simulink model "band_pass_filter_cosim"  (Simulink 6.0)
settings: Solver=ode45  StartTime=0.0  StopTime=0.35  RelTol=1e-3
undefined symbols (not defined in the file): sigbuilder_block
libraries: aldec_ahdl x6
settings Model: LastModifiedBy=arekg

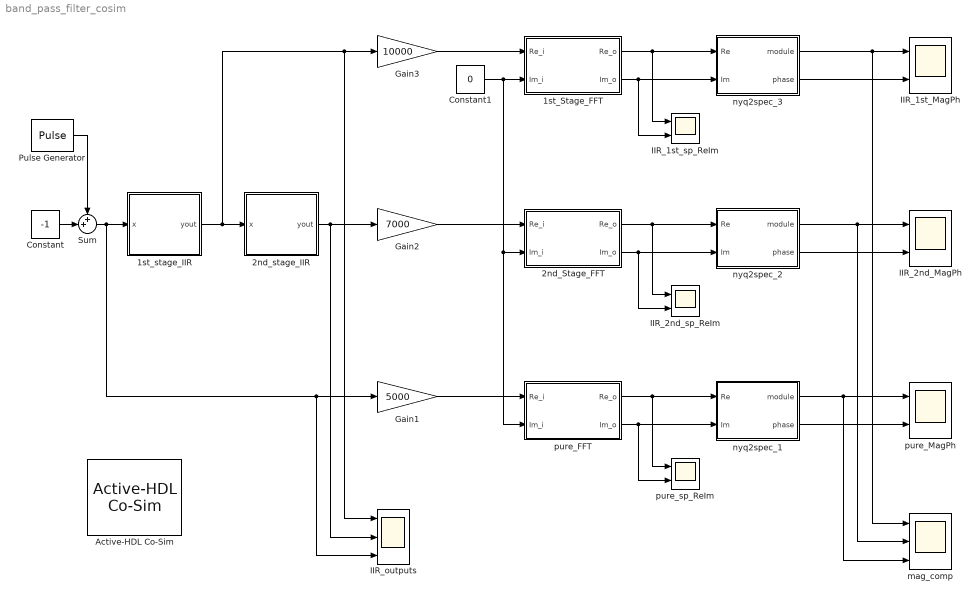
== system band_pass_filter_cosim ==
  1st_Stage_FFT : Subsystem
  1st_stage_IIR : Subsystem
  2nd_Stage_FFT : Subsystem
  2nd_stage_IIR : Subsystem
  Active-HDL Co-Sim : aldec_ahdl/Active-HDL Co-Sim  b_type=0  sys_period=1/88000  dbg=off  quit_en=off  gen_tb=off  tb_fn=mlab_post_tb.log
  Constant : Constant  Value=-1
  Constant1 : Constant  Value=0
  Gain1 : Gain  Gain=5000
  Gain2 : Gain  Gain=7000
  Gain3 : Gain  Gain=10000
  IIR_1st_MagPh : Scope  NumInputPorts=2
      settings: TimeRange=0.35  YMin=0~-4  YMax=80000~4  SaveName=ScopeData8
  IIR_1st_sp_ReIm : Scope  NumInputPorts=2
      settings: TimeRange=0.35  YMin=-80000~-15000  YMax=40000~15000  SaveName=ScopeData9
  IIR_2nd_MagPh : Scope  NumInputPorts=2
      settings: TimeRange=0.35  YMin=0~-4  YMax=90000~4
  IIR_2nd_sp_ReIm : Scope  NumInputPorts=2
      settings: TimeRange=0.35  YMin=-40000~-25000  YMax=80000~25000
  IIR_outputs : Scope  NumInputPorts=3
      settings: TimeRange=0.004173519736842107  YMin=-1~-1~-1  YMax=1~1~1  SaveName=ScopeData6
  Pulse Generator : DiscretePulseGenerator  PulseType=Time based  Amplitude=2  Period=1/1000  PulseWidth=50
  Sum : Sum  Inputs=++|
  mag_comp : Scope  NumInputPorts=3
      settings: TimeRange=0.35  YMin=0~0~0  YMax=80000~90000~70000  SaveName=ScopeData5
  nyq2spec_1 : Subsystem
  nyq2spec_2 : Subsystem
  nyq2spec_3 : Subsystem
  pure_FFT : Subsystem
  pure_MagPh : Scope  NumInputPorts=2
      settings: TimeRange=0.35  YMin=0~-4  YMax=70000~4  SaveName=ScopeData3
  pure_sp_ReIm : Scope  NumInputPorts=2
      settings: TimeRange=0.35  YMin=-60000~-25  YMax=80000~20  SaveName=ScopeData4
  wires:
  1st_stage_IIR/1(yout) -> Gain3/1, IIR_outputs/1, 2nd_stage_IIR/1(x)
  Sum/1 -> 1st_stage_IIR/1(x), Gain1/1, IIR_outputs/3
  2nd_Stage_FFT/1(Re_o) -> IIR_2nd_sp_ReIm/1, nyq2spec_2/1(Re)
  2nd_Stage_FFT/2(Im_o) -> IIR_2nd_sp_ReIm/2, nyq2spec_2/2(Im)
  nyq2spec_2/1(module) -> IIR_2nd_MagPh/1, mag_comp/2
  nyq2spec_2/2(phase) -> IIR_2nd_MagPh/2
  pure_FFT/1(Re_o) -> pure_sp_ReIm/1, nyq2spec_1/1(Re)
  pure_FFT/2(Im_o) -> pure_sp_ReIm/2, nyq2spec_1/2(Im)
  nyq2spec_1/1(module) -> pure_MagPh/1, mag_comp/3
  nyq2spec_1/2(phase) -> pure_MagPh/2
  Gain2/1 -> 2nd_Stage_FFT/1(Re_i)
  Gain1/1 -> pure_FFT/1(Re_i)
  2nd_stage_IIR/1(yout) -> Gain2/1, IIR_outputs/2
  Constant1/1 -> 1st_Stage_FFT/2(Im_i), 2nd_Stage_FFT/2(Im_i), pure_FFT/2(Im_i)
  1st_Stage_FFT/1(Re_o) -> IIR_1st_sp_ReIm/1, nyq2spec_3/1(Re)
  1st_Stage_FFT/2(Im_o) -> IIR_1st_sp_ReIm/2, nyq2spec_3/2(Im)
  nyq2spec_3/1(module) -> IIR_1st_MagPh/1, mag_comp/1
  nyq2spec_3/2(phase) -> IIR_1st_MagPh/2
  Gain3/1 -> 1st_Stage_FFT/1(Re_i)
  Constant/1 -> Sum/2
  Pulse Generator/1 -> Sum/1

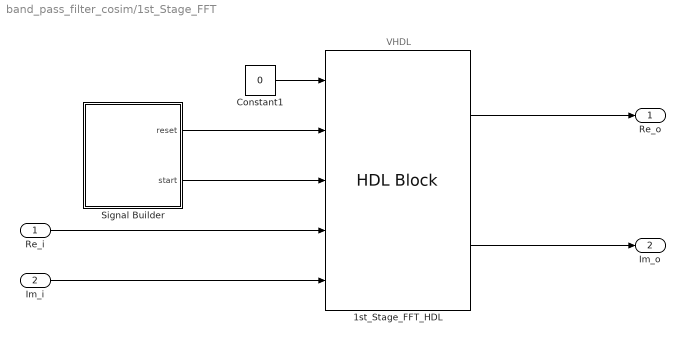
== system band_pass_filter_cosim/1st_Stage_FFT ==
  note: VHDL
  Re_i : Inport  Port=1  LatchInput=off
  Im_i : Inport  Port=2  LatchInput=off
  1st_Stage_FFT_HDL : aldec_ahdl/HDL Block  module_m=top_fft_top_fft  b_type=0  sample=1/22000  mode=Enabled  dbg=off
  Constant1 : Constant  Value=0
  Signal Builder : Subsystem  Tag=STV Subsys  LoadFcn=sigbuilder_block('load');  StartFcn=sigbuilder_block('start');  StopFcn=sigbuilder_block('stop');  ClipboardFcn=sigbuilder_block('clipboard');  mask(Sigbuilder block){}
      mask help: Sigbuilder GUI
      mask init:
      | if ~strcmp(get_param(bdroot(gcb),'SimulationStatus'),'stopped') tuvar = sigbuilder_block('maskInit'); end
      settings: CopyFcn=sigbuilder_block('copy');  DeleteFcn=sigbuilder_block('delete');  ModelCloseFcn=sigbuilder_block('modelClose');  PreSaveFcn=sigbuilder_block('preSave');  NameChangeFcn=sigbuilder_block('namechange');  OpenFcn=sigbuilder_block('open',[102 45 572.25 398.25 ]);  CloseFcn=sigbuilder_block('close');
      mask Display: plot(0,0,100,100,[10,10,40,40,10],[80,20,20,80,80],[40,10],[50,50], [40,27,10],[65,72,56],[40,25,25,10],[28,28,43,43]);
  Re_o : Outport
  Im_o : Outport  Port=2
  wires:
  Re_i/1 -> 1st_Stage_FFT_HDL/4
  Im_i/1 -> 1st_Stage_FFT_HDL/5
  Constant1/1 -> 1st_Stage_FFT_HDL/1
  Signal Builder/2(start) -> 1st_Stage_FFT_HDL/3
  Signal Builder/1(reset) -> 1st_Stage_FFT_HDL/2
  1st_Stage_FFT_HDL/1 -> Re_o/1
  1st_Stage_FFT_HDL/2 -> Im_o/1

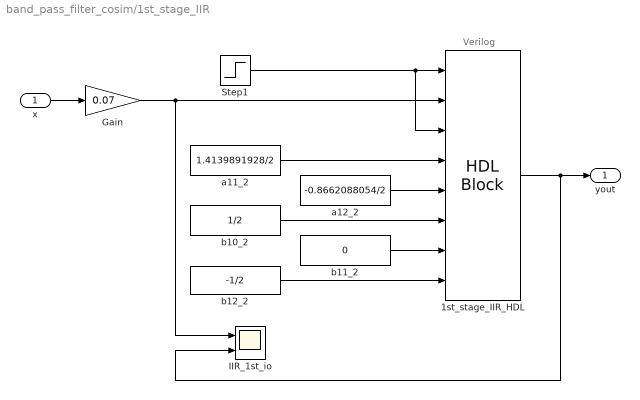
== system band_pass_filter_cosim/1st_stage_IIR ==
  note: Verilog
  x : Inport  Port=1  LatchInput=off
  1st_stage_IIR_HDL : aldec_ahdl/HDL Block  module_m=biquad  b_type=0  sample=1/44000  mode=Enabled  dbg=off
  Gain : Gain  Gain=0.07  SaturateOnIntegerOverflow=on
  IIR_1st_io : Scope  NumInputPorts=2
      settings: TimeRange=0.006433823529411766  YMin=-0.08~-1  YMax=0.08~1  SaveName=ScopeData2
  Step1 : Step  Time=1/22000  SampleTime=1/22000
  a11_2 : Constant  Value=1.4139891928/2
  a12_2 : Constant  Value=-0.8662088054/2
  b10_2 : Constant  Value=1/2
  b11_2 : Constant  Value=0
  b12_2 : Constant  Value=-1/2
  yout : Outport
  wires:
  x/1 -> Gain/1
  Gain/1 -> IIR_1st_io/1, 1st_stage_IIR_HDL/2
  b12_2/1 -> 1st_stage_IIR_HDL/8
  b10_2/1 -> 1st_stage_IIR_HDL/6
  a12_2/1 -> 1st_stage_IIR_HDL/5
  a11_2/1 -> 1st_stage_IIR_HDL/4
  b11_2/1 -> 1st_stage_IIR_HDL/7
  Step1/1 -> 1st_stage_IIR_HDL/1, 1st_stage_IIR_HDL/3
  1st_stage_IIR_HDL/1 -> yout/1, IIR_1st_io/2

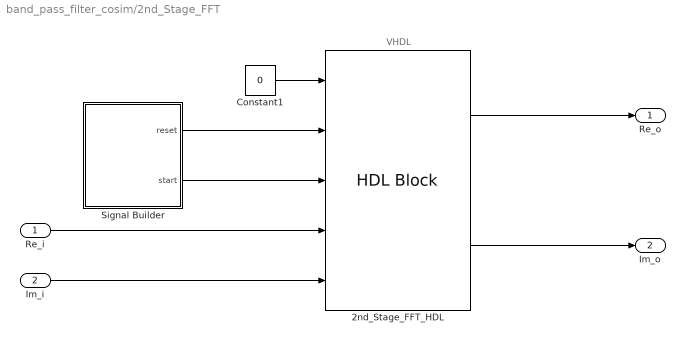
== system band_pass_filter_cosim/2nd_Stage_FFT ==
  note: VHDL
  Re_i : Inport  Port=1  LatchInput=off
  Im_i : Inport  Port=2  LatchInput=off
  2nd_Stage_FFT_HDL : aldec_ahdl/HDL Block  module_m=top_fft_top_fft  b_type=0  sample=1/22000  mode=Enabled  dbg=off
  Constant1 : Constant  Value=0
  Signal Builder : Subsystem  Tag=STV Subsys  LoadFcn=sigbuilder_block('load');  StartFcn=sigbuilder_block('start');  StopFcn=sigbuilder_block('stop');  ClipboardFcn=sigbuilder_block('clipboard');  mask(Sigbuilder block){}
      mask help: Sigbuilder GUI
      mask init:
      | if ~strcmp(get_param(bdroot(gcb),'SimulationStatus'),'stopped') tuvar = sigbuilder_block('maskInit'); end
      settings: CopyFcn=sigbuilder_block('copy');  DeleteFcn=sigbuilder_block('delete');  ModelCloseFcn=sigbuilder_block('modelClose');  PreSaveFcn=sigbuilder_block('preSave');  NameChangeFcn=sigbuilder_block('namechange');  OpenFcn=sigbuilder_block('open',[102 45 572.25 398.25 ]);  CloseFcn=sigbuilder_block('close');
      mask Display: plot(0,0,100,100,[10,10,40,40,10],[80,20,20,80,80],[40,10],[50,50], [40,27,10],[65,72,56],[40,25,25,10],[28,28,43,43]);
  Re_o : Outport
  Im_o : Outport  Port=2
  wires:
  Re_i/1 -> 2nd_Stage_FFT_HDL/4
  Im_i/1 -> 2nd_Stage_FFT_HDL/5
  Constant1/1 -> 2nd_Stage_FFT_HDL/1
  Signal Builder/2(start) -> 2nd_Stage_FFT_HDL/3
  Signal Builder/1(reset) -> 2nd_Stage_FFT_HDL/2
  2nd_Stage_FFT_HDL/1 -> Re_o/1
  2nd_Stage_FFT_HDL/2 -> Im_o/1

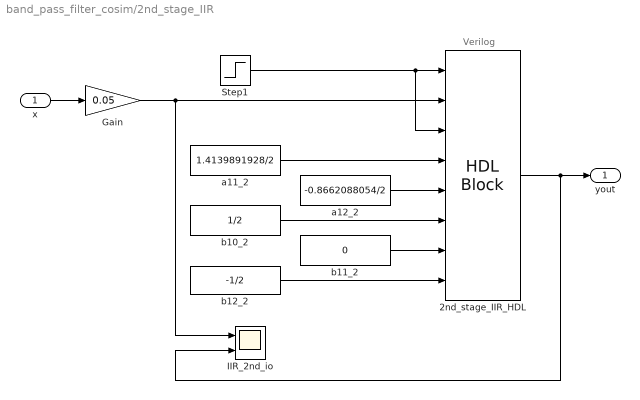
== system band_pass_filter_cosim/2nd_stage_IIR ==
  note: Verilog
  x : Inport  Port=1  LatchInput=off
  2nd_stage_IIR_HDL : aldec_ahdl/HDL Block  module_m=biquad  b_type=0  sample=1/44000  mode=Enabled  dbg=off
  Gain : Gain  Gain=0.05  SaturateOnIntegerOverflow=on
  IIR_2nd_io : Scope  NumInputPorts=2
      settings: TimeRange=0.006433823529411766  YMin=-0.08~-1  YMax=0.08~1  SaveName=ScopeData7
  Step1 : Step  Time=1/22000  SampleTime=1/22000
  a11_2 : Constant  Value=1.4139891928/2
  a12_2 : Constant  Value=-0.8662088054/2
  b10_2 : Constant  Value=1/2
  b11_2 : Constant  Value=0
  b12_2 : Constant  Value=-1/2
  yout : Outport
  wires:
  x/1 -> Gain/1
  Gain/1 -> 2nd_stage_IIR_HDL/2, IIR_2nd_io/1
  b12_2/1 -> 2nd_stage_IIR_HDL/8
  b10_2/1 -> 2nd_stage_IIR_HDL/6
  a12_2/1 -> 2nd_stage_IIR_HDL/5
  a11_2/1 -> 2nd_stage_IIR_HDL/4
  b11_2/1 -> 2nd_stage_IIR_HDL/7
  Step1/1 -> 2nd_stage_IIR_HDL/1, 2nd_stage_IIR_HDL/3
  2nd_stage_IIR_HDL/1 -> yout/1, IIR_2nd_io/2

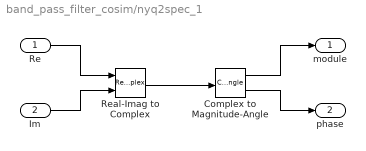
== system band_pass_filter_cosim/nyq2spec_1 ==
  Re : Inport  Port=1  LatchInput=off
  Im : Inport  Port=2  LatchInput=off
  Complex to Magnitude-Angle : ComplexToMagnitudeAngle
  Real-Imag to Complex : RealImagToComplex
  module : Outport
  phase : Outport  Port=2
  wires:
  Re/1 -> Real-Imag to Complex/1
  Real-Imag to Complex/1 -> Complex to Magnitude-Angle/1
  Complex to Magnitude-Angle/1 -> module/1
  Im/1 -> Real-Imag to Complex/2
  Complex to Magnitude-Angle/2 -> phase/1

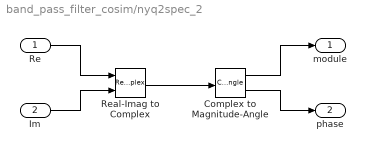
== system band_pass_filter_cosim/nyq2spec_2 ==
  Re : Inport  Port=1  LatchInput=off
  Im : Inport  Port=2  LatchInput=off
  Complex to Magnitude-Angle : ComplexToMagnitudeAngle
  Real-Imag to Complex : RealImagToComplex
  module : Outport
  phase : Outport  Port=2
  wires:
  Re/1 -> Real-Imag to Complex/1
  Real-Imag to Complex/1 -> Complex to Magnitude-Angle/1
  Complex to Magnitude-Angle/1 -> module/1
  Im/1 -> Real-Imag to Complex/2
  Complex to Magnitude-Angle/2 -> phase/1

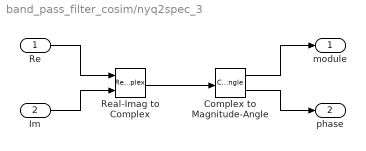
== system band_pass_filter_cosim/nyq2spec_3 ==
  Re : Inport  Port=1  LatchInput=off
  Im : Inport  Port=2  LatchInput=off
  Complex to Magnitude-Angle : ComplexToMagnitudeAngle
  Real-Imag to Complex : RealImagToComplex
  module : Outport
  phase : Outport  Port=2
  wires:
  Re/1 -> Real-Imag to Complex/1
  Real-Imag to Complex/1 -> Complex to Magnitude-Angle/1
  Complex to Magnitude-Angle/1 -> module/1
  Im/1 -> Real-Imag to Complex/2
  Complex to Magnitude-Angle/2 -> phase/1

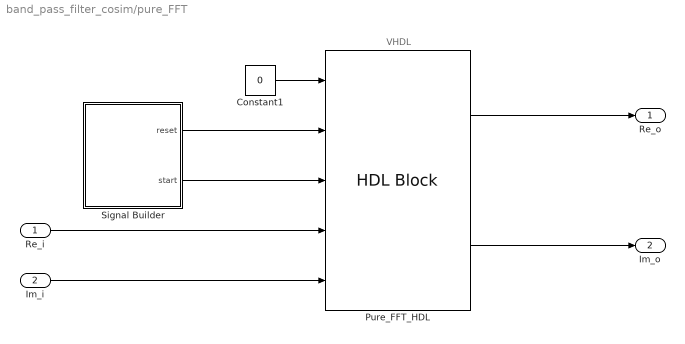
== system band_pass_filter_cosim/pure_FFT ==
  note: VHDL
  Re_i : Inport  Port=1  LatchInput=off
  Im_i : Inport  Port=2  LatchInput=off
  Constant1 : Constant  Value=0
  Pure_FFT_HDL : aldec_ahdl/HDL Block  module_m=top_fft_top_fft  b_type=0  sample=1/22000  mode=Enabled  dbg=off
  Signal Builder : Subsystem  Tag=STV Subsys  LoadFcn=sigbuilder_block('load');  StartFcn=sigbuilder_block('start');  StopFcn=sigbuilder_block('stop');  ClipboardFcn=sigbuilder_block('clipboard');  mask(Sigbuilder block){}
      mask help: Sigbuilder GUI
      mask init:
      | if ~strcmp(get_param(bdroot(gcb),'SimulationStatus'),'stopped') tuvar = sigbuilder_block('maskInit'); end
      settings: CopyFcn=sigbuilder_block('copy');  DeleteFcn=sigbuilder_block('delete');  ModelCloseFcn=sigbuilder_block('modelClose');  PreSaveFcn=sigbuilder_block('preSave');  NameChangeFcn=sigbuilder_block('namechange');  OpenFcn=sigbuilder_block('open',[102 45 572.25 398.25 ]);  CloseFcn=sigbuilder_block('close');
      mask Display: plot(0,0,100,100,[10,10,40,40,10],[80,20,20,80,80],[40,10],[50,50], [40,27,10],[65,72,56],[40,25,25,10],[28,28,43,43]);
  Re_o : Outport
  Im_o : Outport  Port=2
  wires:
  Re_i/1 -> Pure_FFT_HDL/4
  Im_i/1 -> Pure_FFT_HDL/5
  Constant1/1 -> Pure_FFT_HDL/1
  Signal Builder/2(start) -> Pure_FFT_HDL/3
  Signal Builder/1(reset) -> Pure_FFT_HDL/2
  Pure_FFT_HDL/1 -> Re_o/1
  Pure_FFT_HDL/2 -> Im_o/1

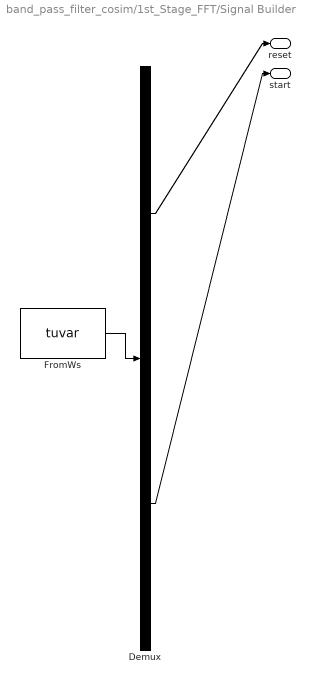
== system band_pass_filter_cosim/1st_Stage_FFT/Signal Builder ==
  Demux : Demux  Tag=STV Demux  Outputs=2
  FromWs : FromWorkspace  Tag=STV FromWs  VariableName=tuvar  SampleTime=1.1364e-005  OutputAfterFinalValue=Holding final value  SigBuilderData=DataTag0
      SigBuilderData=|
      | channels(1).label = 'reset'
      | channels(1).allXData = {[0 0.000318182 0.000318182 0.0227272727273]}
      | channels(1).allYData = {[1 1 0 0]}
      | channels(2).label = 'start'
      | channels(2).allXData = {[0 0.000363636 0.000363636 0.000409091 0.000409091 0.0227272727273]}
      | channels(2).allYData = {[0 0 1 1 0 0]}
      | common.afterFinalStr = 'Hold final value'
      | common.sampleTime = 1.13636363636e-05
      | dataSet.timeRange = [0 0.0227272727273]
      | dataSet.name = 'Group 1'
  reset : Outport  Tag=STV Outport
  start : Outport  Tag=STV Outport  Port=2
  wires:
  FromWs/1 -> Demux/1
  Demux/1 -> reset/1
  Demux/2 -> start/1

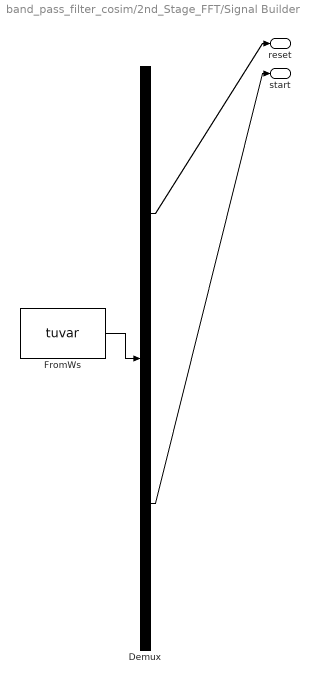
== system band_pass_filter_cosim/2nd_Stage_FFT/Signal Builder ==
  Demux : Demux  Tag=STV Demux  Outputs=2
  FromWs : FromWorkspace  Tag=STV FromWs  VariableName=tuvar  SampleTime=1.1364e-005  OutputAfterFinalValue=Holding final value  SigBuilderData=DataTag1
      SigBuilderData=|
      | channels(1).label = 'reset'
      | channels(1).allXData = {[0 0.000318182 0.000318182 0.0227272727273]}
      | channels(1).allYData = {[1 1 0 0]}
      | channels(2).label = 'start'
      | channels(2).allXData = {[0 0.000363636 0.000363636 0.000409091 0.000409091 0.0227272727273]}
      | channels(2).allYData = {[0 0 1 1 0 0]}
      | common.afterFinalStr = 'Hold final value'
      | common.sampleTime = 1.13636363636e-05
      | dataSet.timeRange = [0 0.0227272727273]
      | dataSet.name = 'Group 1'
  reset : Outport  Tag=STV Outport
  start : Outport  Tag=STV Outport  Port=2
  wires:
  FromWs/1 -> Demux/1
  Demux/1 -> reset/1
  Demux/2 -> start/1

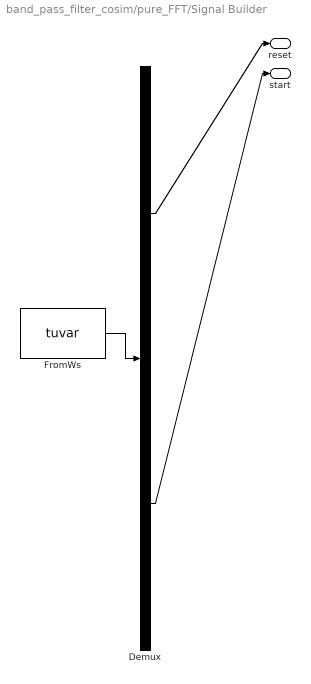
== system band_pass_filter_cosim/pure_FFT/Signal Builder ==
  Demux : Demux  Tag=STV Demux  Outputs=2
  FromWs : FromWorkspace  Tag=STV FromWs  VariableName=tuvar  SampleTime=1.1364e-005  OutputAfterFinalValue=Holding final value  SigBuilderData=DataTag2
      SigBuilderData=|
      | channels(1).label = 'reset'
      | channels(1).allXData = {[0 0.000318182 0.000318182 0.0227272727273]}
      | channels(1).allYData = {[1 1 0 0]}
      | channels(2).label = 'start'
      | channels(2).allXData = {[0 0.000363636 0.000363636 0.000409091 0.000409091 0.0227272727273]}
      | channels(2).allYData = {[0 0 1 1 0 0]}
      | common.afterFinalStr = 'Hold final value'
      | common.sampleTime = 1.13636363636e-05
      | dataSet.timeRange = [0 0.0227272727273]
      | dataSet.name = 'Group 1'
  reset : Outport  Tag=STV Outport
  start : Outport  Tag=STV Outport  Port=2
  wires:
  FromWs/1 -> Demux/1
  Demux/1 -> reset/1
  Demux/2 -> start/1
